simulink model "EMI_SC01A_Finite_Edge"  (R2026a)
settings: Solver=ode23t  StopTime=5.0000000000000004e-06  MaxStep=1e-9  RelTol=1e-6  AbsTol=1e-9
model workspace (MAT data in the model file):
  sc01aCurrentCommutation = timeseries
  sc01aCurrentCommutation.Name = 'unnamed'
  sc01aCurrentCommutation.DataInfo = tsdata.datametadata
  sc01aCurrentCommutation.DataInfo.Interpolation = tsdata.interpolation
  sc01aCurrentCommutation.DataInfo.Interpolation.Fhandle : function handle (value not decoded)
  sc01aCurrentCommutation.DataInfo.Interpolation.Name = 'linear'
  sc01aCurrentCommutation.TimeInfo = tsdata.timemetadata
  sc01aCurrentCommutation.TimeInfo.Length = 5
  sc01aCurrentCommutation.TimeInfo.DuplicateTimes = 0
  sc01aCurrentCommutation.TimeInfo.Time_ = [0; 1e-06; 1.1e-06; 1.2e-06; 5e-06]
  sc01aCurrentCommutation.TimeInfo.Initialized = 1
  sc01aCurrentCommutation.QualityInfo = tsdata.qualmetadata
  sc01aCurrentCommutation.Data_ = [0; 0; 1.5; 3; 3]
  sc01aInducedNegative = [0  0; 1e-06  0; 1e-06  0.255; 1.1e-06  0.255; 1.1e-06  0.255; 1.2e-06  0.255; 1.2e-06  0; 5e-06  0; 5e-06  0]
  sc01aInducedPositive = [0  0; 1e-06  0; 1e-06  0.3; 1.1e-06  0.3; 1.1e-06  0.3; 1.2e-06  0.3; 1.2e-06  0; 5e-06  0; 5e-06  0]
  sc01aParams.meta.id = "SC01A-ASSUMED-V1"
  sc01aParams.meta.provenance = "Assumed circuit and prescribed test excitations; no selected hardware or measurements"
  sc01aParams.source.voltageStep_V = 24
  sc01aParams.source.currentStep_A = 3
  sc01aParams.source.voltageRise_s = 1e-07
  sc01aParams.source.currentRise_s = 2e-07
  sc01aParams.source.edgeTime_s = 1e-06
  sc01aParams.source.pwmFrequency_Hz = 20000
  sc01aParams.source.duty = 0.5
  sc01aParams.driver.commonMode_V = 2.5
  sc01aParams.driver.differential_V = 2
  sc01aParams.driver.transitionTime_s = 1e-07
  sc01aParams.driver.Rp_Ohm = 47
  sc01aParams.driver.Rn_Ohm = 53
  sc01aParams.receiver.Rdiff_Ohm = 120
  sc01aParams.receiver.Cdiff_F = 1e-10
  sc01aParams.receiver.Cp_F = 5e-11
  sc01aParams.receiver.Cn_F = 7e-11
  sc01aParams.receiver.RpBias_Ohm = 10000
  sc01aParams.receiver.RnBias_Ohm = 20000
  sc01aParams.coupling.Cp_F = 1e-11
  sc01aParams.coupling.Cn_F = 9e-12
  sc01aParams.coupling.Mp_H = 2e-08
  sc01aParams.coupling.Mn_H = 1.7e-08
  sc01aParams.ground.R_Ohm = 0.025
  sc01aParams.ground.L_H = 2e-08
  sc01aParams.diagnostics.noiseThreshold_V = 0.2
  sc01aParams.diagnostics.receiverThreshold_V = 0.2
  sc01aParams.diagnostics.commonModeLimit_V = 7
  sc01aParams.simulation.singleStop_s = 5e-06
  sc01aParams.verification.relativeGate = 0.01
  sc01aParams.verification.voltageFloor_V = 0.0001
  sc01aParams.verification.timeGate_s = 1e-09
  sc01aSourceNegative = timeseries
  sc01aSourceNegative.Name = 'unnamed'
  sc01aSourceNegative.DataInfo = tsdata.datametadata
  sc01aSourceNegative.DataInfo.Interpolation = tsdata.interpolation
  sc01aSourceNegative.DataInfo.Interpolation.Fhandle : function handle (value not decoded)
  sc01aSourceNegative.DataInfo.Interpolation.Name = 'linear'
  sc01aSourceNegative.TimeInfo = tsdata.timemetadata
  sc01aSourceNegative.TimeInfo.Length = 5
  sc01aSourceNegative.TimeInfo.DuplicateTimes = 0
  sc01aSourceNegative.TimeInfo.Time_ = [0; 1e-06; 1.1e-06; 1.2e-06; 5e-06]
  sc01aSourceNegative.TimeInfo.Initialized = 1
  sc01aSourceNegative.QualityInfo = tsdata.qualmetadata
  sc01aSourceNegative.Data_ = [1.5; 1.5; 1.5; 1.5; 1.5]
  sc01aSourcePositive = timeseries
  sc01aSourcePositive.Name = 'unnamed'
  sc01aSourcePositive.DataInfo = tsdata.datametadata
  sc01aSourcePositive.DataInfo.Interpolation = tsdata.interpolation
  sc01aSourcePositive.DataInfo.Interpolation.Fhandle : function handle (value not decoded)
  sc01aSourcePositive.DataInfo.Interpolation.Name = 'linear'
  sc01aSourcePositive.TimeInfo = tsdata.timemetadata
  sc01aSourcePositive.TimeInfo.Length = 5
  sc01aSourcePositive.TimeInfo.DuplicateTimes = 0
  sc01aSourcePositive.TimeInfo.Time_ = [0; 1e-06; 1.1e-06; 1.2e-06; 5e-06]
  sc01aSourcePositive.TimeInfo.Initialized = 1
  sc01aSourcePositive.QualityInfo = tsdata.qualmetadata
  sc01aSourcePositive.Data_ = [3.5; 3.5; 3.5; 3.5; 3.5]
  sc01aTopology.schema = 5
  sc01aTopology.positiveCoupling = 1
  sc01aTopology.negativeCoupling = 1
  sc01aVoltageAggressor = timeseries
  sc01aVoltageAggressor.Name = 'unnamed'
  sc01aVoltageAggressor.DataInfo = tsdata.datametadata
  sc01aVoltageAggressor.DataInfo.Interpolation = tsdata.interpolation
  sc01aVoltageAggressor.DataInfo.Interpolation.Fhandle : function handle (value not decoded)
  sc01aVoltageAggressor.DataInfo.Interpolation.Name = 'linear'
  sc01aVoltageAggressor.TimeInfo = tsdata.timemetadata
  sc01aVoltageAggressor.TimeInfo.Length = 5
  sc01aVoltageAggressor.TimeInfo.DuplicateTimes = 0
  sc01aVoltageAggressor.TimeInfo.Time_ = [0; 1e-06; 1.1e-06; 1.2e-06; 5e-06]
  sc01aVoltageAggressor.TimeInfo.Initialized = 1
  sc01aVoltageAggressor.QualityInfo = tsdata.qualmetadata
  sc01aVoltageAggressor.Data_ = [0; 0; 24; 24; 24]
  sc01aVoltageAggressorDerivative = [0  0; 1e-06  0; 1e-06  240000000; 1.1e-06  240000000; 1.1e-06  0; 1.2e-06  0; 1.2e-06  0; 5e-06  0; 5e-06  0]
libraries: fl_lib x23, nesl_utility x11
settings Model: Creator=adand  LastModifiedBy=adand

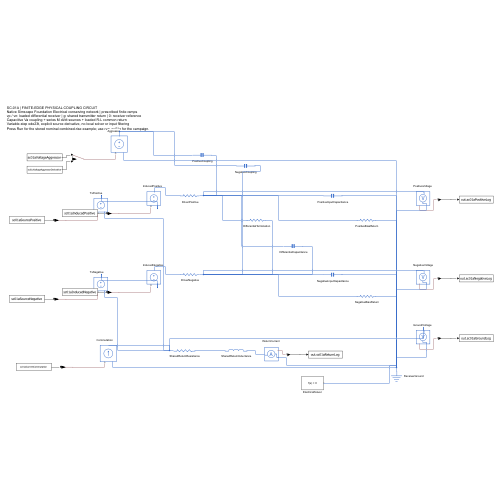
[thumbnail: Simulink's stored preview of the top-level diagram]
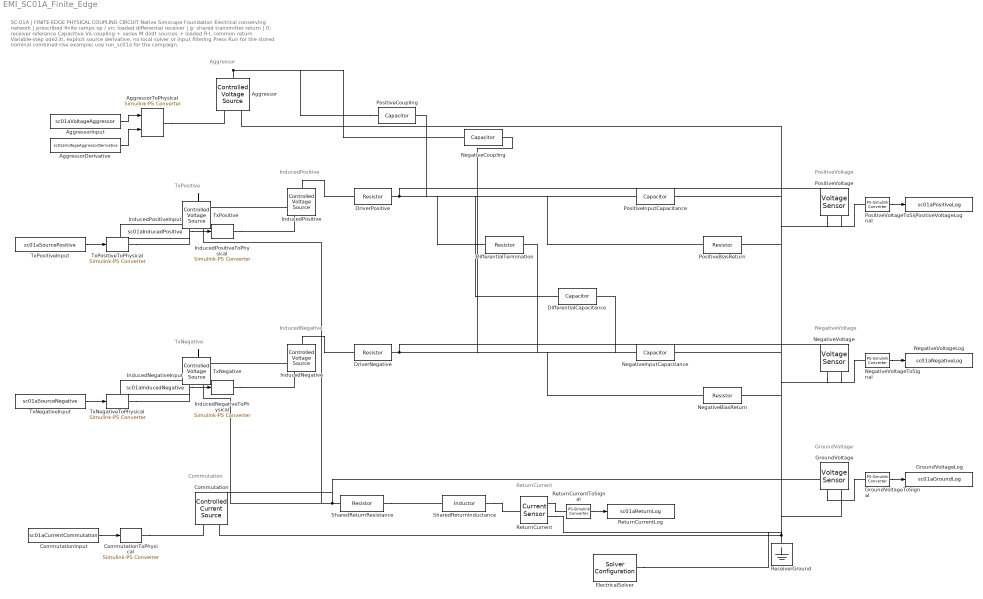
== system EMI_SC01A_Finite_Edge ==
  note: Aggressor
  note: TxPositive
  note: InducedPositive
  note: TxNegative
  note: InducedNegative
  note: Commutation
  note: PositiveVoltage
  note: NegativeVoltage
  note: GroundVoltage
  note: ReturnCurrent
  note: SC-01A | FINITE-EDGE PHYSICAL COUPLING CIRCUIT
      | Native Simscape Foundation Electrical conserving network | prescribed finite ramps
      | vp / vn: loaded differential receiver | g: shared transmitter return | 0: receiver reference
      | Capacitive Va coupling + series M di/dt sources + loaded R-L common return
      | Variable-step ode23t, explicit source derivative, no local solver or input filtering
      | Press Run for the stored nominal combined-rise example; use run_sc01a for the campaign.
  Aggressor : fl_lib/Electrical/Electrical Sources/Controlled Voltage Source
  AggressorDerivative : FromWorkspace  VariableName=sc01aVoltageAggressorDerivative  OutputAfterFinalValue=Holding final value
  AggressorInput : FromWorkspace  VariableName=sc01aVoltageAggressor  OutputAfterFinalValue=Holding final value
  AggressorToPhysical : nesl_utility/Simulink-PS Converter  PhysicalDomain=network_engine_domain  SubClassName=ps_input  LeftPortType=input  RightPortType=output  PseudoPeriodic=off  Frequencies=[]  NoiseDistribution=none  NoiseParameters=[]  Unit=V  AffineConversion=off  FilteringAndDerivatives=provide  SimscapeFilterOrder=1  InputFilterTimeConstant=0.001  UdotUserProvided=1
  Commutation : fl_lib/Electrical/Electrical Sources/Controlled Current Source
  CommutationInput : FromWorkspace  VariableName=sc01aCurrentCommutation  OutputAfterFinalValue=Holding final value
  CommutationToPhysical : nesl_utility/Simulink-PS Converter  PhysicalDomain=network_engine_domain  SubClassName=ps_input  LeftPortType=input  RightPortType=output  PseudoPeriodic=off  Frequencies=[]  NoiseDistribution=none  NoiseParameters=[]  Unit=A  AffineConversion=off  FilteringAndDerivatives=provide  SimscapeFilterOrder=1  InputFilterTimeConstant=0.001  UdotUserProvided=0
  DifferentialCapacitance : fl_lib/Electrical/Electrical Elements/Capacitor  c=sc01aParams.receiver.Cdiff_F F  r=0 Ohm  g=0 1/Ohm  i_specify=off  i_priority=None  i=0 A  i_nominal_specify=off  i_nominal_value=1  i_nominal_unit=A  v_specify=off  v_priority=None  v=0 V  v_nominal_specify=off  v_nominal_value=1  v_nominal_unit=V  vc_specify=off  vc_priority=High  vc=0 V  vc_nominal_specify=off  vc_nominal_value=1  vc_nominal_unit=V
  DifferentialTermination : fl_lib/Electrical/Electrical Elements/Resistor  R=sc01aParams.receiver.Rdiff_Ohm Ohm  i_specify=off  i_priority=None  i=0 A  i_nominal_specify=off  i_nominal_value=1  i_nominal_unit=A  v_specify=off  v_priority=None  v=0 V  v_nominal_specify=off  v_nominal_value=1  v_nominal_unit=V
  DriverNegative : fl_lib/Electrical/Electrical Elements/Resistor  R=sc01aParams.driver.Rn_Ohm Ohm  i_specify=off  i_priority=None  i=0 A  i_nominal_specify=off  i_nominal_value=1  i_nominal_unit=A  v_specify=off  v_priority=None  v=0 V  v_nominal_specify=off  v_nominal_value=1  v_nominal_unit=V
  DriverPositive : fl_lib/Electrical/Electrical Elements/Resistor  R=sc01aParams.driver.Rp_Ohm Ohm  i_specify=off  i_priority=None  i=0 A  i_nominal_specify=off  i_nominal_value=1  i_nominal_unit=A  v_specify=off  v_priority=None  v=0 V  v_nominal_specify=off  v_nominal_value=1  v_nominal_unit=V
  ElectricalSolver : nesl_utility/Solver Configuration  PhysicalDomain=network_engine_domain  SubClassName=solver  LeftPortType=input  RightPortType=generic  Tones=[]  Harmonics=[]  SimulateNoise=off  Profile=off  UseLocalSampling=off  EnableSwitchedLinearOptims=on  FrequencyDomain=off  UseCCode=off  RelTol=0.001  AbsTol=0.001  MinStep=1e-09  ToWorkspace=off  RevertToSquareIcSolve=off  NumHomotopyIterations=100  PhasorMode=off  PhasorModeNumHarmonics=1  ConsistencySolver=NEWTON_XTOL_AFTER_FTOL  CanonicalOrdering=CANONICAL  OptimizeIntermediates=OPTIMIZED  IndexReductionMethod=DerivativeReplacement  DoDC=on  ResidualTolerance=1e-09  ConsistencyTolSource=GLOBAL  ConsistencyAbsTol=0.001  ConsistencyRelTol=0.001  ConsistencyTolFactor=0.001  UseLocalSolver=off  LocalSolverChoice=NE_BACKWARD_EULER_ADVANCER  ResolveIndetEquations=on  FunctionEvalNumThread=1  LocalSolverSampleTime=0.001  DoFixedCost=off  MaxNonlinIter=3  MaxModeIter=2  ComputeImpulses=off  ImpulseIterations=2  LinearAlgebra=auto  LinearAlgebraNumThread=0  EquationFormulation=NE_TIME_EF  DelaysMemoryBudget=1024  AutomaticFiltering=off  FilteringTimeConstant=0.001  PartitionStorageMethod=AS_NEEDED  PartitionMemoryBudget=1024  PartitionMethod=ROBUST  MultibodyUseLocalSolver=off  MultibodyLocalSolverChoice=ODE1  MultibodyLocalSolverSampleTime=0.001
  GroundVoltage : fl_lib/Electrical/Electrical Sensors/Voltage Sensor
  GroundVoltageLog : ToWorkspace  VariableName=sc01aGroundLog  SaveFormat=Timeseries  SampleTime=-1
  GroundVoltageToSignal : nesl_utility/PS-Simulink Converter  PhysicalDomain=network_engine_domain  SubClassName=ps_output  LeftPortType=input  RightPortType=output  PseudoPeriodic=off  Frequencies=[]  VectorFormat=inherit  Unit=V  AffineConversion=off
  InducedNegative : fl_lib/Electrical/Electrical Sources/Controlled Voltage Source
  InducedNegativeInput : FromWorkspace  VariableName=sc01aInducedNegative  OutputAfterFinalValue=Holding final value
  InducedNegativeToPhysical : nesl_utility/Simulink-PS Converter  PhysicalDomain=network_engine_domain  SubClassName=ps_input  LeftPortType=input  RightPortType=output  PseudoPeriodic=off  Frequencies=[]  NoiseDistribution=none  NoiseParameters=[]  Unit=V  AffineConversion=off  FilteringAndDerivatives=provide  SimscapeFilterOrder=1  InputFilterTimeConstant=0.001  UdotUserProvided=0
  InducedPositive : fl_lib/Electrical/Electrical Sources/Controlled Voltage Source
  InducedPositiveInput : FromWorkspace  VariableName=sc01aInducedPositive  OutputAfterFinalValue=Holding final value
  InducedPositiveToPhysical : nesl_utility/Simulink-PS Converter  PhysicalDomain=network_engine_domain  SubClassName=ps_input  LeftPortType=input  RightPortType=output  PseudoPeriodic=off  Frequencies=[]  NoiseDistribution=none  NoiseParameters=[]  Unit=V  AffineConversion=off  FilteringAndDerivatives=provide  SimscapeFilterOrder=1  InputFilterTimeConstant=0.001  UdotUserProvided=0
  NegativeBiasReturn : fl_lib/Electrical/Electrical Elements/Resistor  R=sc01aParams.receiver.RnBias_Ohm Ohm  i_specify=off  i_priority=None  i=0 A  i_nominal_specify=off  i_nominal_value=1  i_nominal_unit=A  v_specify=off  v_priority=None  v=0 V  v_nominal_specify=off  v_nominal_value=1  v_nominal_unit=V
  NegativeCoupling : fl_lib/Electrical/Electrical Elements/Capacitor  c=sc01aParams.coupling.Cn_F F  r=0 Ohm  g=0 1/Ohm  i_specify=off  i_priority=None  i=0 A  i_nominal_specify=off  i_nominal_value=1  i_nominal_unit=A  v_specify=off  v_priority=None  v=0 V  v_nominal_specify=off  v_nominal_value=1  v_nominal_unit=V  vc_specify=off  vc_priority=High  vc=0 V  vc_nominal_specify=off  vc_nominal_value=1  vc_nominal_unit=V
  NegativeInputCapacitance : fl_lib/Electrical/Electrical Elements/Capacitor  c=sc01aParams.receiver.Cn_F F  r=0 Ohm  g=0 1/Ohm  i_specify=off  i_priority=None  i=0 A  i_nominal_specify=off  i_nominal_value=1  i_nominal_unit=A  v_specify=off  v_priority=None  v=0 V  v_nominal_specify=off  v_nominal_value=1  v_nominal_unit=V  vc_specify=off  vc_priority=High  vc=0 V  vc_nominal_specify=off  vc_nominal_value=1  vc_nominal_unit=V
  NegativeVoltage : fl_lib/Electrical/Electrical Sensors/Voltage Sensor
  NegativeVoltageLog : ToWorkspace  VariableName=sc01aNegativeLog  SaveFormat=Timeseries  SampleTime=-1
  NegativeVoltageToSignal : nesl_utility/PS-Simulink Converter  PhysicalDomain=network_engine_domain  SubClassName=ps_output  LeftPortType=input  RightPortType=output  PseudoPeriodic=off  Frequencies=[]  VectorFormat=inherit  Unit=V  AffineConversion=off
  PositiveBiasReturn : fl_lib/Electrical/Electrical Elements/Resistor  R=sc01aParams.receiver.RpBias_Ohm Ohm  i_specify=off  i_priority=None  i=0 A  i_nominal_specify=off  i_nominal_value=1  i_nominal_unit=A  v_specify=off  v_priority=None  v=0 V  v_nominal_specify=off  v_nominal_value=1  v_nominal_unit=V
  PositiveCoupling : fl_lib/Electrical/Electrical Elements/Capacitor  c=sc01aParams.coupling.Cp_F F  r=0 Ohm  g=0 1/Ohm  i_specify=off  i_priority=None  i=0 A  i_nominal_specify=off  i_nominal_value=1  i_nominal_unit=A  v_specify=off  v_priority=None  v=0 V  v_nominal_specify=off  v_nominal_value=1  v_nominal_unit=V  vc_specify=off  vc_priority=High  vc=0 V  vc_nominal_specify=off  vc_nominal_value=1  vc_nominal_unit=V
  PositiveInputCapacitance : fl_lib/Electrical/Electrical Elements/Capacitor  c=sc01aParams.receiver.Cp_F F  r=0 Ohm  g=0 1/Ohm  i_specify=off  i_priority=None  i=0 A  i_nominal_specify=off  i_nominal_value=1  i_nominal_unit=A  v_specify=off  v_priority=None  v=0 V  v_nominal_specify=off  v_nominal_value=1  v_nominal_unit=V  vc_specify=off  vc_priority=High  vc=0 V  vc_nominal_specify=off  vc_nominal_value=1  vc_nominal_unit=V
  PositiveVoltage : fl_lib/Electrical/Electrical Sensors/Voltage Sensor
  PositiveVoltageLog : ToWorkspace  VariableName=sc01aPositiveLog  SaveFormat=Timeseries  SampleTime=-1
  PositiveVoltageToSignal : nesl_utility/PS-Simulink Converter  PhysicalDomain=network_engine_domain  SubClassName=ps_output  LeftPortType=input  RightPortType=output  PseudoPeriodic=off  Frequencies=[]  VectorFormat=inherit  Unit=V  AffineConversion=off
  ReceiverGround : fl_lib/Electrical/Electrical Elements/Electrical Reference
  ReturnCurrent : fl_lib/Electrical/Electrical Sensors/Current Sensor
  ReturnCurrentLog : ToWorkspace  VariableName=sc01aReturnLog  SaveFormat=Timeseries  SampleTime=-1
  ReturnCurrentToSignal : nesl_utility/PS-Simulink Converter  PhysicalDomain=network_engine_domain  SubClassName=ps_output  LeftPortType=input  RightPortType=output  PseudoPeriodic=off  Frequencies=[]  VectorFormat=inherit  Unit=A  AffineConversion=off
  SharedReturnInductance : fl_lib/Electrical/Electrical Elements/Inductor  l=sc01aParams.ground.L_H H  r=0 Ohm  g=0 1/Ohm  i_specify=off  i_priority=None  i=0 A  i_nominal_specify=off  i_nominal_value=1  i_nominal_unit=A  v_specify=off  v_priority=None  v=0 V  v_nominal_specify=off  v_nominal_value=1  v_nominal_unit=V  i_L_specify=off  i_L_priority=High  i_L=0 A  i_L_nominal_specify=off  i_L_nominal_value=1  i_L_nominal_unit=A
  SharedReturnResistance : fl_lib/Electrical/Electrical Elements/Resistor  R=sc01aParams.ground.R_Ohm Ohm  i_specify=off  i_priority=None  i=0 A  i_nominal_specify=off  i_nominal_value=1  i_nominal_unit=A  v_specify=off  v_priority=None  v=0 V  v_nominal_specify=off  v_nominal_value=1  v_nominal_unit=V
  TxNegative : fl_lib/Electrical/Electrical Sources/Controlled Voltage Source
  TxNegativeInput : FromWorkspace  VariableName=sc01aSourceNegative  OutputAfterFinalValue=Holding final value
  TxNegativeToPhysical : nesl_utility/Simulink-PS Converter  PhysicalDomain=network_engine_domain  SubClassName=ps_input  LeftPortType=input  RightPortType=output  PseudoPeriodic=off  Frequencies=[]  NoiseDistribution=none  NoiseParameters=[]  Unit=V  AffineConversion=off  FilteringAndDerivatives=provide  SimscapeFilterOrder=1  InputFilterTimeConstant=0.001  UdotUserProvided=0
  TxPositive : fl_lib/Electrical/Electrical Sources/Controlled Voltage Source
  TxPositiveInput : FromWorkspace  VariableName=sc01aSourcePositive  OutputAfterFinalValue=Holding final value
  TxPositiveToPhysical : nesl_utility/Simulink-PS Converter  PhysicalDomain=network_engine_domain  SubClassName=ps_input  LeftPortType=input  RightPortType=output  PseudoPeriodic=off  Frequencies=[]  NoiseDistribution=none  NoiseParameters=[]  Unit=V  AffineConversion=off  FilteringAndDerivatives=provide  SimscapeFilterOrder=1  InputFilterTimeConstant=0.001  UdotUserProvided=0
  wires:
  AggressorDerivative/1 -> AggressorToPhysical/2
  AggressorInput/1 -> AggressorToPhysical/1
  TxPositiveInput/1 -> TxPositiveToPhysical/1
  InducedPositiveInput/1 -> InducedPositiveToPhysical/1
  TxNegativeInput/1 -> TxNegativeToPhysical/1
  InducedNegativeInput/1 -> InducedNegativeToPhysical/1
  CommutationInput/1 -> CommutationToPhysical/1
  PositiveVoltageToSignal/1 -> PositiveVoltageLog/1
  NegativeVoltageToSignal/1 -> NegativeVoltageLog/1
  GroundVoltageToSignal/1 -> GroundVoltageLog/1
  ReturnCurrentToSignal/1 -> ReturnCurrentLog/1
  connections:
  AggressorToPhysical/RConn1 -- Aggressor/RConn1
  TxPositiveToPhysical/RConn1 -- TxPositive/RConn1
  InducedPositiveToPhysical/RConn1 -- InducedPositive/RConn1
  TxNegativeToPhysical/RConn1 -- TxNegative/RConn1
  InducedNegativeToPhysical/RConn1 -- InducedNegative/RConn1
  CommutationToPhysical/RConn1 -- Commutation/RConn1
  PositiveVoltage/RConn1 -- PositiveVoltageToSignal/LConn1
  NegativeVoltage/RConn1 -- NegativeVoltageToSignal/LConn1
  GroundVoltage/RConn1 -- GroundVoltageToSignal/LConn1
  ReturnCurrent/RConn1 -- ReturnCurrentToSignal/LConn1
  Aggressor/RConn2 -- ReceiverGround/LConn1 -- Commutation/RConn2 -- PositiveInputCapacitance/RConn1 -- PositiveBiasReturn/RConn1 -- NegativeInputCapacitance/RConn1 -- NegativeBiasReturn/RConn1 -- ReturnCurrent/RConn2 -- ElectricalSolver/RConn1 -- PositiveVoltage/RConn2 -- NegativeVoltage/RConn2 -- GroundVoltage/RConn2
  TxPositive/RConn2 -- SharedReturnResistance/LConn1 -- TxNegative/RConn2 -- Commutation/LConn1 -- GroundVoltage/LConn1
  TxPositive/LConn1 -- InducedPositive/RConn2
  InducedPositive/LConn1 -- DriverPositive/LConn1
  TxNegative/LConn1 -- InducedNegative/RConn2
  InducedNegative/LConn1 -- DriverNegative/LConn1
  PositiveCoupling/LConn1 -- Aggressor/LConn1 -- NegativeCoupling/LConn1
  PositiveCoupling/RConn1 -- DriverPositive/RConn1 -- DifferentialTermination/LConn1 -- DifferentialCapacitance/LConn1 -- PositiveInputCapacitance/LConn1 -- PositiveBiasReturn/LConn1 -- PositiveVoltage/LConn1
  NegativeCoupling/RConn1 -- DriverNegative/RConn1 -- DifferentialTermination/RConn1 -- DifferentialCapacitance/RConn1 -- NegativeInputCapacitance/LConn1 -- NegativeBiasReturn/LConn1 -- NegativeVoltage/LConn1
  SharedReturnResistance/RConn1 -- SharedReturnInductance/LConn1
  SharedReturnInductance/RConn1 -- ReturnCurrent/LConn1
